simulink model "simulink_bode_draw"  (R2016a)
settings: Solver=VariableStepAuto  StartTime=0.0  StopTime=10.0  RelTol=1e-3
settings Model: Creator=xlh  LastModifiedBy=xlh

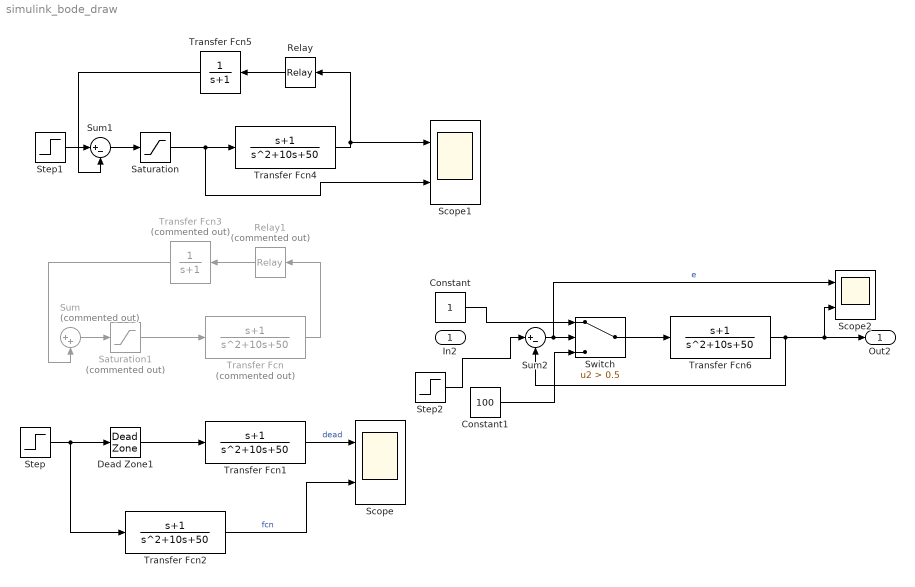
== system simulink_bode_draw ==
  In2 : Inport
  Constant : Constant
  Constant1 : Constant  Value=100
  Dead Zone1 : DeadZone  SaturateOnIntegerOverflow=on
  Relay : Relay
  Relay1 : Relay  Commented=on
  Saturation : Saturate  UpperLimit=1  LowerLimit=-1
  Saturation1 : Saturate  Commented=on  UpperLimit=1  LowerLimit=-1
  Scope : Scope  NumInputPorts=2
  Scope1 : Scope  NumInputPorts=2
  Scope2 : Scope  NumInputPorts=2
  Step : Step  SampleTime=0
  Step1 : Step  Time=2  SampleTime=0
  Step2 : Step  SampleTime=0
  Sum : Sum  Commented=on  Inputs=|++
  Sum1 : Sum  Inputs=|+-
  Sum2 : Sum  Inputs=|+-
  Switch : Switch  Criteria=u2 > Threshold  Threshold=0.5
  Transfer Fcn : TransferFcn  Commented=on  Numerator=[1 1]  Denominator=[1 10 50]
  Transfer Fcn{1..2,4,6} (4 alike) : TransferFcn  Numerator=[1 1]  Denominator=[1 10 50]
  Transfer Fcn3 : TransferFcn  Commented=on  Denominator=[1 1]
  Transfer Fcn5 : TransferFcn  Denominator=[1 1]
  Out2 : Outport
  wires:
  Transfer Fcn/1 -> Relay1/1
  Saturation1/1 -> Transfer Fcn/1
  Transfer Fcn1/1 -> Scope/1  "dead"
  Step/1 -> Transfer Fcn2/1, Dead Zone1/1
  Dead Zone1/1 -> Transfer Fcn1/1
  Transfer Fcn2/1 -> Scope/2  "fcn"
  Relay1/1 -> Transfer Fcn3/1
  Sum/1 -> Saturation1/1
  Transfer Fcn3/1 -> Sum/2
  Transfer Fcn4/1 -> Relay/1, Scope1/1
  Saturation/1 -> Scope1/2, Transfer Fcn4/1
  Relay/1 -> Transfer Fcn5/1
  Step1/1 -> Sum1/1
  Sum1/1 -> Saturation/1
  Transfer Fcn5/1 -> Sum1/2
  Transfer Fcn6/1 -> Sum2/2, Scope2/2, Out2/1
  Sum2/1 -> Scope2/1, Switch/2  "e"
  Switch/1 -> Transfer Fcn6/1
  Constant1/1 -> Switch/3
  Constant/1 -> Switch/1
  Step2/1 -> Sum2/1
